simulink model "discrete_continuous"  (R2019a)
settings: Solver=ode4  StartTime=0.0  StopTime=10.0  FixedStep=0.001  RelTol=1e-3
settings Model: Creator=crs20  LastModifiedBy=crs20

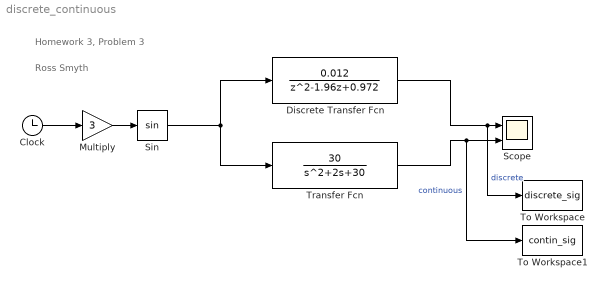
== system discrete_continuous ==
  note: Ross Smyth
  note: Homework 3, Problem 3
  Clock : Clock
      settings: Decimation=1000
  Discrete Transfer Fcn : DiscreteTransferFcn  Numerator=[0.012]  Denominator=[1 -1.96 0.972]  SampleTime=0.02
  Multiply : Gain  Gain=3
  Scope : Scope  NumInputPorts=2
  Sin : Trigonometry
  To Workspace : ToWorkspace  VariableName=discrete_sig  SaveFormat=Timeseries  SampleTime=0.001
  To Workspace1 : ToWorkspace  VariableName=contin_sig  SaveFormat=Timeseries  SampleTime=-1
  Transfer Fcn : TransferFcn  Numerator=[30]  Denominator=[1 2 30]
  wires:
  Clock/1 -> Multiply/1
  Sin/1 -> Transfer Fcn/1, Discrete Transfer Fcn/1
  Multiply/1 -> Sin/1
  Discrete Transfer Fcn/1 -> To Workspace/1, Scope/1  "discrete"
  Transfer Fcn/1 -> To Workspace1/1, Scope/2  "continuous"
